simulink model "MEMS_Switch"  (R2018b)
settings: Solver=VariableStepAuto  StartTime=0.0  StopTime=40e-6  FixedStep=1e-6  MaxStep=0.1e-6  RelTol=1e-3
values from neighbouring files (symbols this model uses):
  g0 = 3e-6    (= 3e-06)    [F_Contact.m]    (also in F_Electrostatic.m; Pulse_MEMS.m; Qe_Factor.m; Run_MEMS_Sim.m)
  k = 10.0    (= 10)    [F_Contact.m]    (also in F_Electrostatic.m; Pulse_MEMS.m; Qe_Factor.m; Run_MEMS_Sim.m)
  m = 0.35*(w)*(l)*(t)*(19320)    (= 1.62288e-10)    [F_Contact.m]    (also in F_Electrostatic.m; Pulse_MEMS.m; Qe_Factor.m; Run_MEMS_Sim.m)
  V = 42    [F_Contact.m]    (also in F_Electrostatic.m; Pulse_MEMS.m; Qe_Factor.m; Run_MEMS_Sim.m = 30)
settings Model: Creator=njcoburn  LastModifiedBy=stange
settings DataIOCC: ReturnWorkspaceOutputs=on

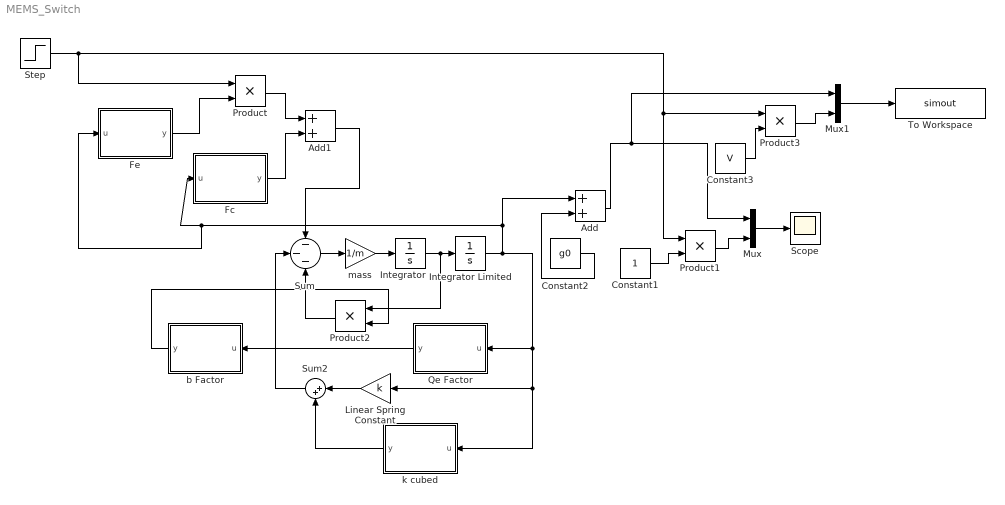
== system MEMS_Switch ==
  Add : Sum
  Add1 : Sum
  Constant1 : Constant
  Constant2 : Constant  Value=g0
  Constant3 : Constant  Value=V
  Fc : MATLAB Function  TreatAsAtomicUnit=on
  Fe : MATLAB Function  TreatAsAtomicUnit=on
  Integrator : Integrator  ZeroCross=off
  Integrator Limited : Integrator  UpperSaturationLimit=g0  AbsoluteTolerance=1e-9  ZeroCross=off
  Linear Spring Constant : Gain  Gain=k
  Mux : Mux  Inputs=2
  Mux1 : Mux  Inputs=2
  Product{,1..3} (4 alike) : Product
  Qe Factor : MATLAB Function  TreatAsAtomicUnit=on
  Scope : Scope
  Step : Step  Time=50e-6  Before=1  After=0  SampleTime=0
  Sum : Sum  Inputs=---
  Sum2 : Sum  Inputs=|++
  To Workspace : ToWorkspace  VariableName=simout  SaveFormat=Timeseries  SampleTime=-1
  b Factor : MATLAB Function  TreatAsAtomicUnit=on
  k cubed : MATLAB Function  TreatAsAtomicUnit=on
  mass : Gain  Gain=1/m
  wires:
  Sum/1 -> mass/1
  mass/1 -> Integrator/1
  Integrator/1 -> Product2/1, Integrator Limited/1
  Linear Spring Constant/1 -> Sum2/1
  k cubed/1(y) -> Sum2/2
  Sum2/1 -> Sum/2
  Constant1/1 -> Product1/2
  Mux/1 -> Scope/1
  Product1/1 -> Mux/2
  Product2/1 -> Sum/3
  Step/1 -> Product/1, Product1/1, Product3/1
  Fe/1(y) -> Product/2
  Qe Factor/1(y) -> b Factor/1(u)
  b Factor/1(y) -> Product2/2
  Product/1 -> Add1/1
  Fc/1(y) -> Add1/2
  Add1/1 -> Sum/1
  Integrator Limited/1 -> Qe Factor/1(u), Linear Spring Constant/1, k cubed/1(u), Add/1, Fe/1(u), Fc/1(u)
  Add/1 -> Mux1/1, Mux/1
  Constant2/1 -> Add/2
  Mux1/1 -> To Workspace/1
  Product3/1 -> Mux1/2
  Constant3/1 -> Product3/2

== matlab function MEMS_Switch/Fc ==
  data: u input; y output
function y = fcn(u)
%#codegen
coder.extrinsic('evalin', 'assignin')

C1 = 0;                  % Needed in order to set variable class correctly
C1 = evalin('base','C1'); % Read value from workspace

C2 = 0;                  % Needed in order to set variable class correctly
C2 = evalin('base','C2'); % Read value from workspace

A = 0;                  % Needed in order to set variable class correctly
A = evalin('base','A'); % Read value from workspace

g0 = 0;                  % Needed in order to set variable class correctly
g0 = evalin('base','g0'); % Read value from workspace

y = C1*A/((g0+u)^3)-C2*A/((g0+u)^10);

== matlab function MEMS_Switch/Fe ==
  data: u input; y output
function y = fcn(u)
%#codegen
coder.extrinsic('evalin', 'assignin')

g0 = 0;                  % Needed in order to set variable class correctly
g0 = evalin('base','g0'); % Read value from workspace

t_d = 0;                  % Needed in order to set variable class correctly
t_d = evalin('base','t_d'); % Read value from workspace

e_r = 0;                  % Needed in order to set variable class correctly
e_r = evalin('base','e_r'); % Read value from workspace

e0 = 0;                  % Needed in order to set variable class correctly
e0 = evalin('base','e0'); % Read value from workspace

A = 0;                  % Needed in order to set variable class correctly
A = evalin('base','A'); % Read value from workspace

V = 0;                  % Needed in order to set variable class correctly
V = evalin('base','V'); % Read value from workspace

y = .5*e0*A*(V^2)/(((g0+(t_d/e_r)+u))^2);

== matlab function MEMS_Switch/Qe Factor ==
  data: u input; y output
function y = fcn(u)
%#codegen
coder.extrinsic('evalin', 'assignin')

Q = 0;                  % Needed in order to set variable class correctly
Q = evalin('base','Q'); % Read value from workspace

g0 = 0;                  % Needed in order to set variable class correctly
g0 = evalin('base','g0'); % Read value from workspace

y_x = 0;                  % Needed in order to set variable class correctly
y_x = evalin('base','y_x'); % Read value from workspace

y = Q*((1.1-(u/g0)^2))^(1.5)*(1+9.638*((y_x/(g0-u))^1.159));

== matlab function MEMS_Switch/b Factor ==
  data: u input; y output
function y = fcn(u)
%#codegen
coder.extrinsic('evalin', 'assignin')

k = 0;                  % Needed in order to set variable class correctly
k = evalin('base','k'); % Read value from workspace

freq = 0;                  % Needed in order to set variable class correctly
freq = evalin('base','freq'); % Read value from workspace

y = (k/(2*pi*freq*u));

== matlab function MEMS_Switch/k cubed ==
  data: u input; y output
function y = fcn(u)
%#codegen
coder.extrinsic('evalin', 'assignin')

ks = 0;                  % Needed in order to set variable class correctly
ks = evalin('base','ks'); % Read value from workspace

y = (ks)*(u^3);
